simulink model "OPENXWD"  (R2022b)
settings: Solver=ode45  StartTime=0.0  StopTime=inf  RelTol=1e-3  EnableMultiTasking=on
PreLoadFcn:
  | run('Parameters\FSE_Parameters.m')
model workspace (MAT data in the model file):
  socvcb : containers.Map (value not decoded)
undefined symbols (not defined in the file): i_Diff
libraries: CarMaker4SL x21, simulink x16, eeGeneralControl x6
(part 5 of 8)

== system OPENXWD/CarMaker/IPG Vehicle/PowerTrain/Electric Powertrain/E-Gas // E-Motor/Subsystem1/VDC/Vehicle Dynamics Control Modes/VDC Complete/Optimization SKF & CKF ==
  RPM_INV1 : Inport
  RPM_INV2 : Inport  Port=2
  Steer_An : Inport  Port=3
  SKF_Initial : Inport  Port=4
  CKF_Initial : Inport  Port=5
  Cte_SKF : Inport  Port=6
  Cte_CKF : Inport  Port=7
  CKF_prev : DataStoreRead  DataStoreName=B  IndexOptions=Index vector (dialog)  Indices=1  OutputSizes=1
  Constant : Constant  Value=0
  Data Store Memory : DataStoreMemory  ReadBeforeWriteMsg=warning  WriteAfterWriteMsg=warning  WriteAfterReadMsg=warning  ShowAdditionalParam=off
  Data Store Memory1 : DataStoreMemory  DataStoreName=B  ReadBeforeWriteMsg=warning  WriteAfterWriteMsg=warning  WriteAfterReadMsg=warning  ShowAdditionalParam=off
  Data Store Write : DataStoreWrite  IndexOptions=Index vector (dialog)  Indices=1  OutputSizes=1
  Data Store Write1 : DataStoreWrite  DataStoreName=B  IndexOptions=Index vector (dialog)  Indices=1  OutputSizes=1
  Derivative : Derivative
  Display : Display
  Display1 : Display
  Display2 : Display
  MATLAB Function : MATLAB Function  TreatAsAtomicUnit=on
  Mux : Mux  Inputs=3
  "SKF_prev " : DataStoreRead  IndexOptions=Index vector (dialog)  Indices=1  OutputSizes=1
  Saturation : Saturate  UpperLimit=6000  LowerLimit=0
  Scope : Scope
  "Subsystem " : Subsystem
  Switch : Switch  Threshold=900  SaturateOnIntegerOverflow=off  InputSameDT=off
  SKF_act : Outport  VectorParamsAs1DForOutWhenUnconnected=off
  CKF_act : Outport  Port=2  VectorParamsAs1DForOutWhenUnconnected=off
  wires:
  SKF_Initial/1 -> "Subsystem "/3(SKF_Initial)
  CKF_prev/1 -> "Subsystem "/6("CKF_prev ")
  "Subsystem "/1("SKF_act ") -> SKF_act/1, Display1/1, Data Store Write/1  "SKF"
  Derivative/1 -> Switch/1, Switch/2, Saturation/1, Display/1, "Subsystem "/2(Derivative)  "alpha"
  "SKF_prev "/1 -> "Subsystem "/4(SKF_prev)
  "Subsystem "/2(CKF_act) -> CKF_act/1, Display2/1, Data Store Write1/1  "CKF"
  Cte_CKF/1 -> "Subsystem "/8(Cte_CKF)
  Steer_An/1 -> "Subsystem "/1(Steer_An)
  CKF_Initial/1 -> "Subsystem "/5("CKF_Initial ")
  Cte_SKF/1 -> "Subsystem "/7(Cte_SKF)
  MATLAB Function/1(RPM) -> Derivative/1  "w (rad/s)"
  Mux/1 -> Scope/1
  Saturation/1 -> Mux/2
  Switch/1 -> Mux/3
  Constant/1 -> Switch/3
  RPM_INV1/1 -> Mux/1, MATLAB Function/1(RPM_INV1)
  RPM_INV2/1 -> MATLAB Function/2(RPM_INV2)

== system OPENXWD/CarMaker/IPG Vehicle/PowerTrain/Electric Powertrain/E-Gas // E-Motor/Subsystem1/VDC/Vehicle Dynamics Control Modes/VDC Complete/Sensor_DATA ==
  note: [deg]
  note: [N]
  note: [N]
  note: [N]
  note: [N]
  note: [0-1]
  note: [0-1]
  note: [0 or 1]
  note: [rad/s]
  note: [rad/s]
  note: [rad/s]
  note: [m/s2]
  note: [m/s]
  Steer_Ang : Inport
  Ellipse_acc : Inport  Port=2
  Gyro_Ellipse : Inport  Port=3
  FR_Susp : Inport  Port=4
  FL_Susp : Inport  Port=5
  RR_Susp : Inport  Port=6
  RL_Susp : Inport  Port=7
  Gas Pedal : Inport  Port=8
  Brake Pedal : Inport  Port=9
  Regenerative Enable : Inport  Port=10
  V_eRR : Inport  Port=11
  "V_eRL " : Inport  Port=12
  Ellipse_vel : Inport  Port=13
  Steer_ang : Outport  VectorParamsAs1DForOutWhenUnconnected=off
  Ellipse_Acc : Outport  Port=2  VectorParamsAs1DForOutWhenUnconnected=off
  GyroEllipse : Outport  Port=3  VectorParamsAs1DForOutWhenUnconnected=off
  FR_susp : Outport  Port=4  VectorParamsAs1DForOutWhenUnconnected=off
  FL_susp : Outport  Port=5  VectorParamsAs1DForOutWhenUnconnected=off
  RR_susp : Outport  Port=6  VectorParamsAs1DForOutWhenUnconnected=off
  RL_susp : Outport  Port=7  VectorParamsAs1DForOutWhenUnconnected=off
  Gas_Pedal : Outport  Port=8  VectorParamsAs1DForOutWhenUnconnected=off
  Brake_Pedal : Outport  Port=9  VectorParamsAs1DForOutWhenUnconnected=off
  Reg_Enable : Outport  Port=10  VectorParamsAs1DForOutWhenUnconnected=off
  "V_eRR " : Outport  Port=11  VectorParamsAs1DForOutWhenUnconnected=off
  V_eRL : Outport  Port=12  VectorParamsAs1DForOutWhenUnconnected=off
  Ellipse_Vel : Outport  Port=13
  wires:
  RL_Susp/1 -> RL_susp/1
  RR_Susp/1 -> RR_susp/1
  FL_Susp/1 -> FL_susp/1
  FR_Susp/1 -> FR_susp/1
  Steer_Ang/1 -> Steer_ang/1
  Gas Pedal/1 -> Gas_Pedal/1
  Brake Pedal/1 -> Brake_Pedal/1
  Regenerative Enable/1 -> Reg_Enable/1
  "V_eRL "/1 -> V_eRL/1
  V_eRR/1 -> "V_eRR "/1
  Gyro_Ellipse/1 -> GyroEllipse/1
  Ellipse_acc/1 -> Ellipse_Acc/1
  Ellipse_vel/1 -> Ellipse_Vel/1

== system OPENXWD/CarMaker/IPG Vehicle/PowerTrain/Electric Powertrain/E-Gas // E-Motor/Subsystem1/VDC/Vehicle Dynamics Control Modes/VDC Complete/Wheel_to_motor ==
  "Fx_FR " : Inport
  "Fx_FL " : Inport  Port=2
  "Fx_RR " : Inport  Port=3
  "Fx_RL " : Inport  Port=4
  Re : Inport  Port=5
  RT : Inport  Port=6
  Add : Sum  Inputs=+-
  Constant : Constant  Value=0
  Constant1 : Constant  Value=0
  Fx_to_engineTqRL : Subsystem
  Fx_to_engineTqRR : Subsystem
  MATLAB Function1 : MATLAB Function  TreatAsAtomicUnit=on
  MATLAB Function2 : MATLAB Function  TreatAsAtomicUnit=on
  Tq_diff : Outport
  Tq_FR : Outport  Port=2  VectorParamsAs1DForOutWhenUnconnected=off
  Tq_FL : Outport  Port=3  VectorParamsAs1DForOutWhenUnconnected=off
  Tq_RR : Outport  Port=4  VectorParamsAs1DForOutWhenUnconnected=off
  Tq_RL : Outport  Port=5  VectorParamsAs1DForOutWhenUnconnected=off
  wires:
  Fx_to_engineTqRR/1(Tq) -> Add/1, Tq_RR/1
  Fx_to_engineTqRL/1(Tq) -> Tq_RL/1, Add/2
  "Fx_FR "/1 -> Tq_FR/1
  "Fx_FL "/1 -> Tq_FL/1
  Re/1 -> Fx_to_engineTqRR/2(Re), Fx_to_engineTqRL/2(Re)
  RT/1 -> Fx_to_engineTqRR/3(RT), Fx_to_engineTqRL/3(RT)
  "Fx_RL "/1 -> MATLAB Function2/2(v)
  "Fx_RR "/1 -> MATLAB Function1/2(v)
  MATLAB Function2/1(value) -> Fx_to_engineTqRL/1(Fx)
  MATLAB Function1/1(value) -> Fx_to_engineTqRR/1(Fx)
  Constant1/1 -> MATLAB Function1/1(cte)
  Constant/1 -> MATLAB Function2/1(cte)
  Add/1 -> Tq_diff/1

== system OPENXWD/CarMaker/IPG Vehicle/PowerTrain/Electric Powertrain/E-Gas // E-Motor/Subsystem1/VDC/Vehicle Dynamics Control Modes/VDC without Longitudinal/Constraints ==
  Tq_FRin : Inport
  Tq_FLin : Inport  Port=2
  Tq_RR_wc : Inport  Port=3
  "Tq_RL_wc " : Inport  Port=4
  "Trans_max_static " : Inport  Port=5
  Trans_max_dynamic : Inport  Port=6
  V_eRR : Inport  Port=7
  V_eRL : Inport  Port=8
  Tq_max : Inport  Port=9
  MaxRegTorque : Inport  Port=10
  Bp : Inport  Port=11
  Reg_enable : Inport  Port=12
  RT : Inport  Port=13
  Acelerating and braking without Regenerative : Subsystem  TreatAsAtomicUnit=on
  Braking with Regenerative : Subsystem  TreatAsAtomicUnit=on
  Constant : Constant  Value=0
  Constant1 : Constant  Value=0
  If : If  NumInputs=2  IfExpression=u2 == 1 & u1 > 0
  Merge1 : Merge
  Merge2 : Merge
  Tq_FRout : Outport  VectorParamsAs1DForOutWhenUnconnected=off
  "Tq_FLout " : Outport  Port=2  VectorParamsAs1DForOutWhenUnconnected=off
  Tq_RRout : Outport  Port=3  VectorParamsAs1DForOutWhenUnconnected=off
  Tq_RLout : Outport  Port=4  VectorParamsAs1DForOutWhenUnconnected=off
  wires:
  Constant1/1 -> "Tq_FLout "/1
  Constant/1 -> Tq_FRout/1
  Tq_RR_wc/1 -> Acelerating and braking without Regenerative/9(Tq_RR), Braking with Regenerative/2(Tq_RR_wc)
  "Tq_RL_wc "/1 -> Braking with Regenerative/3(Tq_RL_wc), Acelerating and braking without Regenerative/10(Tq_RL)
  Tq_max/1 -> Acelerating and braking without Regenerative/2(Tq_max)
  V_eRL/1 -> Acelerating and braking without Regenerative/4(V_eRL)
  Trans_max_dynamic/1 -> Acelerating and braking without Regenerative/5(Trans_dynamic_max_motor_Tq)
  "Trans_max_static "/1 -> Acelerating and braking without Regenerative/6(Trans_static_max_motor_Tq)
  Merge2/1 -> Tq_RLout/1
  Merge1/1 -> Tq_RRout/1
  Bp/1 -> If/1
  Reg_enable/1 -> If/2
  V_eRR/1 -> Acelerating and braking without Regenerative/3(V_eRR)
  If/1 -> Braking with Regenerative/Action
  If/2 -> Acelerating and braking without Regenerative/Action
  MaxRegTorque/1 -> Braking with Regenerative/1(MaxRegTorque)
  Tq_FRin/1 -> Acelerating and braking without Regenerative/7(Tq_FR)
  Tq_FLin/1 -> Acelerating and braking without Regenerative/8(Tq_FL)
  Acelerating and braking without Regenerative/2(TQ_RL) -> Merge2/1
  Acelerating and braking without Regenerative/1(TQ_RR) -> Merge1/1
  Braking with Regenerative/1(TQ_RR) -> Merge1/2
  Braking with Regenerative/2(TQ_RL) -> Merge2/2
  RT/1 -> Acelerating and braking without Regenerative/1(Transmission Ratio)

== system OPENXWD/CarMaker/IPG Vehicle/PowerTrain/Electric Powertrain/E-Gas // E-Motor/Subsystem1/VDC/Vehicle Dynamics Control Modes/VDC without Longitudinal/Driver // CarBehaviours ==
  Tq_FRin : Inport
  Tq_FLin : Inport  Port=2
  Tq_RRin : Inport  Port=3
  "Tq_RLin " : Inport  Port=4
  Bp : Inport  Port=5
  Ap : Inport  Port=6
  Reg_enable : Inport  Port=7
  Ap_Sat_up : Inport  Port=8
  Ap_Sat_down : Inport  Port=9
  Accelerating : Subsystem  TreatAsAtomicUnit=on
  Braking Conditions : If  NumInputs=4  IfExpression=u1>0.2 & u2<=u4 & u3==1  ElseIfExpressions=u1>0.2 & u2<=u4 & u3==0, u1==0 & u2==0
  Constant : Constant  Value=0
  Constant1 : Constant  Value=0
  Inertia Braking : Subsystem  TreatAsAtomicUnit=on
  Mech_Braking : Subsystem  TreatAsAtomicUnit=on
  Merge : Merge  Inputs=4
  Merge1 : Merge  Inputs=4
  Regenerative+Mech Braking : Subsystem  TreatAsAtomicUnit=on
  Terminator : Terminator
  Terminator1 : Terminator
  Tq_FRout : Outport  VectorParamsAs1DForOutWhenUnconnected=off
  "Tq_FLout " : Outport  Port=2  VectorParamsAs1DForOutWhenUnconnected=off
  Tq_RRout : Outport  Port=3  VectorParamsAs1DForOutWhenUnconnected=off
  Tq_RLout : Outport  Port=4  VectorParamsAs1DForOutWhenUnconnected=off
  out_Throttle : Outport  Port=5  VectorParamsAs1DForOutWhenUnconnected=off
  wires:
  Constant1/1 -> "Tq_FLout "/1
  Constant/1 -> Tq_FRout/1
  Tq_FLin/1 -> Terminator1/1
  Tq_FRin/1 -> Terminator/1
  Merge/1 -> Tq_RRout/1
  Merge1/1 -> Tq_RLout/1
  Bp/1 -> Regenerative+Mech Braking/1(Bp), Braking Conditions/1
  Ap/1 -> Accelerating/1(Ap), Braking Conditions/2
  Regenerative+Mech Braking/1("Tq_RR ") -> Merge/1
  Mech_Braking/1("Tq_RR ") -> Merge/2
  Inertia Braking/1("Tq_RR ") -> Merge/3
  Accelerating/1("Tq_RR ") -> Merge/4
  Regenerative+Mech Braking/2(Tq_RL) -> Merge1/1
  Mech_Braking/2(Tq_RL) -> Merge1/2
  Inertia Braking/2(Tq_RL) -> Merge1/3
  Accelerating/2(Tq_RL) -> Merge1/4
  Braking Conditions/1 -> Regenerative+Mech Braking/Action
  Braking Conditions/2 -> Mech_Braking/Action
  Braking Conditions/3 -> Inertia Braking/Action
  Braking Conditions/4 -> Accelerating/Action
  Tq_RRin/1 -> Regenerative+Mech Braking/2(Tq_max_RR), Accelerating/4(Tq_RR)
  "Tq_RLin "/1 -> Regenerative+Mech Braking/3(Tq_max_RL), Accelerating/5("Tq_RL ")
  Ap_Sat_up/1 -> Accelerating/2("Ap_Sat_up ")
  Ap_Sat_down/1 -> Accelerating/3(Ap_Sat_down), Braking Conditions/4
  Reg_enable/1 -> Braking Conditions/3
  Accelerating/3(Out_Throttle) -> out_Throttle/1

== system OPENXWD/CarMaker/IPG Vehicle/PowerTrain/Electric Powertrain/E-Gas // E-Motor/Subsystem1/VDC/Vehicle Dynamics Control Modes/VDC without Longitudinal/Force to Tq ==
  "Fx_FR " : Inport
  "Fx_FL " : Inport  Port=2
  "Fx_RR " : Inport  Port=3
  "Fx_RL " : Inport  Port=4
  Re : Inport  Port=5
  Constant : Constant  Value=0
  Constant1 : Constant  Value=0
  Fx_to_wheelTqRL : Subsystem
  Fx_to_wheelTqRR : Subsystem
  MATLAB Function1 : MATLAB Function  TreatAsAtomicUnit=on
  MATLAB Function2 : MATLAB Function  TreatAsAtomicUnit=on
  Tq_FR : Outport  VectorParamsAs1DForOutWhenUnconnected=off
  Tq_FL : Outport  Port=2  VectorParamsAs1DForOutWhenUnconnected=off
  Tq_RR : Outport  Port=3  VectorParamsAs1DForOutWhenUnconnected=off
  Tq_RL : Outport  Port=4  VectorParamsAs1DForOutWhenUnconnected=off
  wires:
  Fx_to_wheelTqRR/1(Tq) -> Tq_RR/1
  Fx_to_wheelTqRL/1(Tq) -> Tq_RL/1
  "Fx_FR "/1 -> Tq_FR/1
  "Fx_FL "/1 -> Tq_FL/1
  Re/1 -> Fx_to_wheelTqRR/2(Re), Fx_to_wheelTqRL/2(Re)
  "Fx_RR "/1 -> MATLAB Function2/2(v)
  "Fx_RL "/1 -> MATLAB Function1/2(v)
  MATLAB Function2/1(value) -> Fx_to_wheelTqRR/1(Fx)
  Constant/1 -> MATLAB Function2/1(cte)
  Constant1/1 -> MATLAB Function1/1(cte)
  MATLAB Function1/1(value) -> Fx_to_wheelTqRL/1(Fx)

== system OPENXWD/CarMaker/IPG Vehicle/PowerTrain/Electric Powertrain/E-Gas // E-Motor/Subsystem1/VDC/Vehicle Dynamics Control Modes/VDC without Longitudinal/In_Numbers ==
  C-Kamm_Factor : Inport
  Max Regen Torque [Nm] : Inport  Port=2
  Steering Saturation (per site) [deg] : Inport  Port=3
  Ap_Sat_Down [-] : Inport  Port=4
  Ap_Sat_Up [-] : Inport  Port=5
  3% difference : Gain  Gain=0.97
  Diameter to Radius : Gain  Gain=1/2
  Effective Rolling Diameter[inch] : Constant  Value=18
  Engine+Inverter Performance [-] : Constant  Value=0.8
  Maximum Torque per motor [Nm] : Constant  Value=120
  Maximum Transmission Torque Dynamic [Nm] : Constant  Value=140
  Maximum Transmission Torque Static [Nm] : Constant  Value=130
  Product : Product
  Transmision Ratio[-] : Constant  Value=4
  inch to m : Gain  Gain=0.0254
  Steer_Sat [deg] : Outport  VectorParamsAs1DForOutWhenUnconnected=off
  Tq_Max_Wheel [Nm] : Outport  Port=2  VectorParamsAs1DForOutWhenUnconnected=off
  Cornering Kamm_Factor [0-2] : Outport  Port=3  VectorParamsAs1DForOutWhenUnconnected=off
  Transmision_Ratio[-] : Outport  Port=4  VectorParamsAs1DForOutWhenUnconnected=off
  Effective Rolling Radius[m] : Outport  Port=5  VectorParamsAs1DForOutWhenUnconnected=off
  Ap_Sat_down[-] : Outport  Port=6  VectorParamsAs1DForOutWhenUnconnected=off
  Ap_Sat_up[-] : Outport  Port=7  VectorParamsAs1DForOutWhenUnconnected=off
  Engine+Inverter Performance[-] : Outport  Port=8  VectorParamsAs1DForOutWhenUnconnected=off
  Trans_max _static[Nm] : Outport  Port=9  VectorParamsAs1DForOutWhenUnconnected=off
  Trans_max_dynamic [Nm] : Outport  Port=10  VectorParamsAs1DForOutWhenUnconnected=off
  MaxRegTorque [Nm] : Outport  Port=11  VectorParamsAs1DForOutWhenUnconnected=off
  wires:
  Transmision Ratio[-]/1 -> Product/2, Transmision_Ratio[-]/1
  Effective Rolling Diameter[inch]/1 -> Diameter to Radius/1
  Maximum Transmission Torque Static [Nm]/1 -> Trans_max _static[Nm]/1
  Maximum Transmission Torque Dynamic [Nm]/1 -> Trans_max_dynamic [Nm]/1
  inch to m/1 -> 3% difference/1
  3% difference/1 -> Effective Rolling Radius[m]/1
  Engine+Inverter Performance [-]/1 -> Engine+Inverter Performance[-]/1
  Max Regen Torque [Nm]/1 -> MaxRegTorque [Nm]/1
  C-Kamm_Factor/1 -> Cornering Kamm_Factor [0-2]/1
  Steering Saturation (per site) [deg]/1 -> Steer_Sat [deg]/1
  Ap_Sat_Up [-]/1 -> Ap_Sat_up[-]/1
  Ap_Sat_Down [-]/1 -> Ap_Sat_down[-]/1
  Diameter to Radius/1 -> inch to m/1
  Product/1 -> Tq_Max_Wheel [Nm]/1
  Maximum Torque per motor [Nm]/1 -> Product/1

== system OPENXWD/CarMaker/IPG Vehicle/PowerTrain/Electric Powertrain/E-Gas // E-Motor/Subsystem1/VDC/Vehicle Dynamics Control Modes/VDC without Longitudinal/Kamm Circle Lateral ==
  "N_FR " : Inport
  N_FL : Inport  Port=2
  N_RR : Inport  Port=3
  N_RL : Inport  Port=4
  Fy : Inport  Port=5
  CK_Factor : Inport  Port=6
  Constant : Constant  Value=-1
  Constant1 : Constant  Value=-1
  Kamm_Circle LatD : MATLAB Function  TreatAsAtomicUnit=on
  MATLAB Function1 : MATLAB Function  TreatAsAtomicUnit=on
  MATLAB Function2 : MATLAB Function  TreatAsAtomicUnit=on
  Product : Product
  Product1 : Product
  Fx_FR : Outport  VectorParamsAs1DForOutWhenUnconnected=off
  Fx_FL : Outport  Port=2  VectorParamsAs1DForOutWhenUnconnected=off
  "Fx_RR " : Outport  Port=3  VectorParamsAs1DForOutWhenUnconnected=off
  "Fx_RL " : Outport  Port=4  VectorParamsAs1DForOutWhenUnconnected=off
  wires:
  N_FL/1 -> Fx_FL/1
  "N_FR "/1 -> Fx_FR/1
  N_RL/1 -> Kamm_Circle LatD/2(Fz_L)
  Fy/1 -> Kamm_Circle LatD/3(Fy)
  N_RR/1 -> Kamm_Circle LatD/1(Fz_R)
  Kamm_Circle LatD/1(Fx_R) -> Product/1
  Kamm_Circle LatD/2(Fx_L) -> Product1/1
  CK_Factor/1 -> Product/2, Product1/2
  Product1/1 -> MATLAB Function1/2(v)
  Product/1 -> MATLAB Function2/2(v)
  Constant1/1 -> MATLAB Function2/1(cte)
  Constant/1 -> MATLAB Function1/1(cte)
  MATLAB Function2/1(value) -> "Fx_RR "/1
  MATLAB Function1/1(value) -> "Fx_RL "/1

== system OPENXWD/CarMaker/IPG Vehicle/PowerTrain/Electric Powertrain/E-Gas // E-Motor/Subsystem1/VDC/Vehicle Dynamics Control Modes/VDC without Longitudinal/Lateral Dynamics ==
  FR_susp : Inport
  FL_susp : Inport  Port=2
  RR_susp : Inport  Port=3
  RL_susp : Inport  Port=4
  Gas_pedal : Inport  Port=5
  Brake_pedal : Inport  Port=6
  Ellipse_acc : Inport  Port=7
  Constant : Constant  Value=0
  Constant1 : Constant  Value=0
  Constant2 : Constant  Value=0
  Demux : Demux  Outputs=3
  Fy per wheel : Gain  Gain=1/2
  Gravity : Gain  Gain=1/9.81
  Gravity1 : Gain  Gain=1/9.81
  Product : Product
  Sum : Sum  Inputs=++++
  Sum1 : Sum
  Terminator{3..6} (4 alike) : Terminator
  N_FR : Outport  VectorParamsAs1DForOutWhenUnconnected=off
  "N_FL " : Outport  Port=2  VectorParamsAs1DForOutWhenUnconnected=off
  "N_RR " : Outport  Port=3  VectorParamsAs1DForOutWhenUnconnected=off
  N_RL : Outport  Port=4  VectorParamsAs1DForOutWhenUnconnected=off
  Fy_R : Outport  Port=5  VectorParamsAs1DForOutWhenUnconnected=off
  Mass [kg] (0,inf) : Outport  Port=6  VectorParamsAs1DForOutWhenUnconnected=off
  Handling [-] (-inf,inf) : Outport  Port=7  VectorParamsAs1DForOutWhenUnconnected=off
  wires:
  Constant2/1 -> "N_FL "/1
  Constant1/1 -> N_FR/1
  Gas_pedal/1 -> Terminator4/1
  Brake_pedal/1 -> Terminator5/1
  Demux/2 -> Product/1
  Demux/1 -> Terminator6/1
  Demux/3 -> Terminator3/1
  Product/1 -> Fy per wheel/1  "Fy per axe"
  Fy per wheel/1 -> Fy_R/1
  Gravity1/1 -> Product/2
  Sum/1 -> Gravity/1
  Sum1/1 -> Gravity1/1
  Gravity/1 -> Mass [kg] (0,inf)/1  "Mass [kg]"
  RL_susp/1 -> N_RL/1, Sum1/2, Sum/4
  RR_susp/1 -> Sum1/1, "N_RR "/1, Sum/3
  FL_susp/1 -> Sum/2
  FR_susp/1 -> Sum/1
  Ellipse_acc/1 -> [ellipse_acc]
  Constant/1 -> Handling [-] (-inf,inf)/1
  [ellipse_acc] -> Demux/1

== system OPENXWD/CarMaker/IPG Vehicle/PowerTrain/Electric Powertrain/E-Gas // E-Motor/Subsystem1/VDC/Vehicle Dynamics Control Modes/VDC without Longitudinal/Optimization SKF & CKF ==
  RPM_INV1 : Inport
  RPM_INV2 : Inport  Port=2
  CKF_Initial : Inport  Port=3
  Cte_CKF : Inport  Port=4
  CKF_prev : DataStoreRead  DataStoreName=B  IndexOptions=Index vector (dialog)  Indices=1  OutputSizes=1
  Data Store Memory1 : DataStoreMemory  DataStoreName=B  ReadBeforeWriteMsg=warning  WriteAfterWriteMsg=warning  WriteAfterReadMsg=warning  ShowAdditionalParam=off
  Data Store Write1 : DataStoreWrite  DataStoreName=B  IndexOptions=Index vector (dialog)  Indices=1  OutputSizes=1
  Derivative : Derivative
  MATLAB Function : MATLAB Function  TreatAsAtomicUnit=on
  "Subsystem " : Subsystem
  CKF_act : Outport  VectorParamsAs1DForOutWhenUnconnected=off
  wires:
  CKF_prev/1 -> "Subsystem "/3("CKF_prev ")
  Derivative/1 -> "Subsystem "/1(Derivative)  "alpha"
  MATLAB Function/1(RPM) -> Derivative/1  "w (rad/s)"
  "Subsystem "/1(CKF_act) -> Data Store Write1/1, CKF_act/1  "CKF"
  Cte_CKF/1 -> "Subsystem "/4(Cte_CKF)
  CKF_Initial/1 -> "Subsystem "/2("CKF_Initial ")
  RPM_INV1/1 -> MATLAB Function/1(RPM_INV1)
  RPM_INV2/1 -> MATLAB Function/2(RPM_INV2)

== system OPENXWD/CarMaker/IPG Vehicle/PowerTrain/Electric Powertrain/E-Gas // E-Motor/Subsystem1/VDC/Vehicle Dynamics Control Modes/VDC without Longitudinal/Sensor_DATA ==
  note: [deg]
  note: [N]
  note: [N]
  note: [N]
  note: [N]
  note: [0-1]
  note: [0-1]
  note: [0 or 1]
  note: [rad/s]
  note: [rad/s]
  note: [m/s2]
  Steer_Ang : Inport
  FR_Susp : Inport  Port=2
  FL_Susp : Inport  Port=3
  RR_Susp : Inport  Port=4
  RL_Susp : Inport  Port=5
  Gas Pedal : Inport  Port=6
  Brake Pedal : Inport  Port=7
  Regenerative Enable : Inport  Port=8
  V_eRR : Inport  Port=9
  "V_eRL " : Inport  Port=10
  Ellipse_acc_ax_ay_az : Inport  Port=11
  Steer_ang : Outport  VectorParamsAs1DForOutWhenUnconnected=off
  FR_susp : Outport  Port=2  VectorParamsAs1DForOutWhenUnconnected=off
  FL_susp : Outport  Port=3  VectorParamsAs1DForOutWhenUnconnected=off
  RR_susp : Outport  Port=4  VectorParamsAs1DForOutWhenUnconnected=off
  RL_susp : Outport  Port=5  VectorParamsAs1DForOutWhenUnconnected=off
  Gas_Pedal : Outport  Port=6  VectorParamsAs1DForOutWhenUnconnected=off
  Brake_Pedal : Outport  Port=7  VectorParamsAs1DForOutWhenUnconnected=off
  Reg_Enable : Outport  Port=8  VectorParamsAs1DForOutWhenUnconnected=off
  "V_eRR " : Outport  Port=9  VectorParamsAs1DForOutWhenUnconnected=off
  V_eRL : Outport  Port=10  VectorParamsAs1DForOutWhenUnconnected=off
  Ellipse_acc : Outport  Port=11  VectorParamsAs1DForOutWhenUnconnected=off
  wires:
  RL_Susp/1 -> RL_susp/1
  RR_Susp/1 -> RR_susp/1
  FL_Susp/1 -> FL_susp/1
  FR_Susp/1 -> FR_susp/1
  Steer_Ang/1 -> Steer_ang/1
  Gas Pedal/1 -> Gas_Pedal/1
  Brake Pedal/1 -> Brake_Pedal/1
  Regenerative Enable/1 -> Reg_Enable/1
  "V_eRL "/1 -> V_eRL/1
  V_eRR/1 -> "V_eRR "/1
  Ellipse_acc_ax_ay_az/1 -> Ellipse_acc/1

== system OPENXWD/CarMaker/IPG Vehicle/PowerTrain/Electric Powertrain/E-Gas // E-Motor/Subsystem1/VDC/Vehicle Dynamics Control Modes/Steering TV with TC/Accelerating, Braking or Regen Braking/Accelerating ==
  Throttle : Inport
  Tq_RR : Inport  Port=2
  "Tq_RL " : Inport  Port=3
  Action Port : ActionPort  ActionPortLabel=else
  Product : Product
  Product1 : Product
  "Tq_RR " : Outport  VectorParamsAs1DForOutWhenUnconnected=off
  Tq_RL : Outport  Port=2  VectorParamsAs1DForOutWhenUnconnected=off
  wires:
  Product1/1 -> "Tq_RR "/1
  Product/1 -> Tq_RL/1
  Throttle/1 -> Product/1, Product1/1
  Tq_RR/1 -> Product1/2
  "Tq_RL "/1 -> Product/2

== system OPENXWD/CarMaker/IPG Vehicle/PowerTrain/Electric Powertrain/E-Gas // E-Motor/Subsystem1/VDC/Vehicle Dynamics Control Modes/Steering TV with TC/Accelerating, Braking or Regen Braking/Inertia Braking ==
  Action Port : ActionPort  ActionPortLabel=elseif( u1<=0.2 & u2<=0)
  Constant : Constant  Value=0
  Constant1 : Constant  Value=0
  "Tq_RR " : Outport  VectorParamsAs1DForOutWhenUnconnected=off
  Tq_RL : Outport  Port=2  VectorParamsAs1DForOutWhenUnconnected=off
  wires:
  Constant1/1 -> Tq_RL/1
  Constant/1 -> "Tq_RR "/1

== system OPENXWD/CarMaker/IPG Vehicle/PowerTrain/Electric Powertrain/E-Gas // E-Motor/Subsystem1/VDC/Vehicle Dynamics Control Modes/Steering TV with TC/Accelerating, Braking or Regen Braking/Mech_Braking ==
  Action Port : ActionPort  ActionPortLabel=elseif(u1>0.2 & u2<=0 & u3==0)
  Constant : Constant  Value=0
  Constant1 : Constant  Value=0
  "Tq_RR " : Outport  VectorParamsAs1DForOutWhenUnconnected=off
  Tq_RL : Outport  Port=2  VectorParamsAs1DForOutWhenUnconnected=off
  wires:
  Constant1/1 -> Tq_RL/1
  Constant/1 -> "Tq_RR "/1

== system OPENXWD/CarMaker/IPG Vehicle/PowerTrain/Electric Powertrain/E-Gas // E-Motor/Subsystem1/VDC/Vehicle Dynamics Control Modes/Steering TV with TC/Accelerating, Braking or Regen Braking/Regenerative+Mech Braking ==
  Max_Regen_Tq : Inport
  Bp : Inport  Port=2
  RegTq_RR : Inport  Port=3
  RegTq_RL : Inport  Port=4
  Action Port : ActionPort  ActionPortLabel=if(u1>0.2 & u2<=0 & u3==1)
  Gain : Gain  Gain=-1
  Gain1 : Gain  Gain=-1
  MATLAB Function : MATLAB Function  TreatAsAtomicUnit=on
  MATLAB Function1 : MATLAB Function  TreatAsAtomicUnit=on
  "Tq_RR " : Outport  VectorParamsAs1DForOutWhenUnconnected=off
  Tq_RL : Outport  Port=2  VectorParamsAs1DForOutWhenUnconnected=off
  wires:
  MATLAB Function1/1(RegTq_RR) -> Gain/1
  Gain/1 -> "Tq_RR "/1
  Gain1/1 -> Tq_RL/1
  MATLAB Function1/2(RegTq_RL) -> Gain1/1
  MATLAB Function/2(Tq_regen_RL) -> MATLAB Function1/3(Tq_RL)
  MATLAB Function/1(Tq_regen_RR) -> MATLAB Function1/2(Tq_RR)
  Bp/1 -> MATLAB Function/1(Bp)
  RegTq_RR/1 -> MATLAB Function/2(Tq_max_RR)
  RegTq_RL/1 -> MATLAB Function/3(Tq_max_RL)
  Max_Regen_Tq/1 -> MATLAB Function1/1(MaxRegenTq)

== system OPENXWD/CarMaker/IPG Vehicle/PowerTrain/Electric Powertrain/E-Gas // E-Motor/Subsystem1/VDC/Vehicle Dynamics Control Modes/Steering TV with TC/Optimization SKF & CKF/Subsystem  ==
  Steer_An : Inport
  Derivative : Inport  Port=2
  SKF_Initial : Inport  Port=3
  SKF_prev : Inport  Port=4
  "CKF_Initial " : Inport  Port=5
  "CKF_prev " : Inport  Port=6
  Cte_SKF : Inport  Port=7
  Cte_CKF : Inport  Port=8
  CKF : Subsystem
  MATLAB Function1 : MATLAB Function  TreatAsAtomicUnit=on
  SKF : Subsystem
  SKF or CKF : If  IfExpression=-10 < u1 & u1 < 10
  Steering Wheel Maximum Angle : Constant  Value=100
  "SKF_act " : Outport  VectorParamsAs1DForOutWhenUnconnected=off
  CKF_act : Outport  Port=2  VectorParamsAs1DForOutWhenUnconnected=off
  wires:
  MATLAB Function1/1(value) -> SKF or CKF/1
  Steering Wheel Maximum Angle/1 -> MATLAB Function1/1(cte)
  Steer_An/1 -> MATLAB Function1/2(v)
  SKF/1(SKF_act) -> "SKF_act "/1
  CKF/1("CKF_act ") -> CKF_act/1
  SKF or CKF/1 -> SKF/Action
  SKF or CKF/2 -> CKF/Action
  "CKF_prev "/1 -> CKF/3("CKF_prev ")
  Derivative/1 -> CKF/1(Derivative), SKF/1(Derivative)
  SKF_Initial/1 -> SKF/2("SKF_Initial ")
  SKF_prev/1 -> SKF/3(SKF_prev)
  "CKF_Initial "/1 -> CKF/2(CKF_Initial)
  Cte_SKF/1 -> SKF/4(Cte_SKF)
  Cte_CKF/1 -> CKF/4(Cte_CKF)

== system OPENXWD/CarMaker/IPG Vehicle/PowerTrain/Electric Powertrain/E-Gas // E-Motor/Subsystem1/VDC/Vehicle Dynamics Control Modes/VDC Complete/Constraints and motor to wheel Tq/Acelerating and braking without Regenerative ==
  note: Tq_lim y Flag_Power: antiguamente había aquí la limitación por temperatura y potencia
  Tq_max : Inport
  V_eRR : Inport  Port=2
  V_eRL : Inport  Port=3
  Trans_max_dynamic : Inport  Port=4
  Trans_max_static : Inport  Port=5
  Tq_FR : Inport  Port=6
  Tq_FL : Inport  Port=7
  Tq_RR : Inport  Port=8
  Tq_RL : Inport  Port=9
  Tq_diff : Inport  Port=10
  Tq_diff_max : Inport  Port=11
  Action Port : ActionPort  ActionPortLabel=else
  Constant : Constant  Value=0
  Gain : Gain  Gain=3.141592/30
  If Action 1 : Subsystem  TreatAsAtomicUnit=on
  If Action 2 : Subsystem  TreatAsAtomicUnit=on
  If1 : If  NumInputs=3  IfExpression=u1 > u3 & u2 > u3
  MATLAB Function : MATLAB Function  TreatAsAtomicUnit=on
  Merge2 : Merge
  Momentum Z scaled : Subsystem
  Terminator : Terminator
  Terminator1 : Terminator
  minimum value : MATLAB Function  TreatAsAtomicUnit=on
  minimum value1 : MATLAB Function  TreatAsAtomicUnit=on
  rpm : Constant  Value=200
  TQ_RR : Outport  VectorParamsAs1DForOutWhenUnconnected=off
  TQ_RL : Outport  Port=2  VectorParamsAs1DForOutWhenUnconnected=off
  Flag_Power : Outport  Port=3  VectorParamsAs1DForOutWhenUnconnected=off
  wires:
  If1/1 -> If Action 1/Action
  If Action 1/1(Trans_limit) -> Merge2/1
  Merge2/1 -> minimum value/1(a), minimum value1/1(a)
  Trans_max_dynamic/1 -> If Action 1/1(Trans_max_dynamic)
  If Action 2/1(Trans_limit) -> Merge2/2
  V_eRR/1 -> If1/1
  V_eRL/1 -> If1/2
  If1/2 -> If Action 2/Action
  Trans_max_static/1 -> If Action 2/1("Trans_max_static ")
  Tq_max/1 -> minimum value1/2(b), minimum value/2(b)
  rpm/1 -> Gain/1
  Gain/1 -> If1/3  "approx 20.95"
  Tq_FR/1 -> Terminator/1
  Tq_FL/1 -> Terminator1/1
  Tq_RR/1 -> [tq_RR_wc], minimum value/3(c)
  Tq_RL/1 -> [tq_RL_wc], minimum value1/3(c)
  [tq_RR_wc] -> Momentum Z scaled/3(Tq_RR_wc)
  [tq_RL_wc] -> Momentum Z scaled/4(Tq_RL_wc)
  Momentum Z scaled/1(TQ_RR) -> TQ_RR/1
  Momentum Z scaled/2(TQ_RL) -> TQ_RL/1
  Tq_diff/1 -> MATLAB Function/1(diff_wc)
  Tq_diff_max/1 -> MATLAB Function/2(diff_max)
  MATLAB Function/1(diff_lim) -> [Tq_diff_lim]
  [Tq_diff_lim] -> Momentum Z scaled/5(Tq_diff)
  minimum value/1(min) -> Momentum Z scaled/1(Tq_RR_Lim)
  minimum value1/1(min) -> Momentum Z scaled/2(Tq_RL_Lim)
  Constant/1 -> Flag_Power/1

== system OPENXWD/CarMaker/IPG Vehicle/PowerTrain/Electric Powertrain/E-Gas // E-Motor/Subsystem1/VDC/Vehicle Dynamics Control Modes/VDC Complete/Constraints and motor to wheel Tq/Braking with Regenerative ==
  MaxRegTorque : Inport
  Tq_RR_wc : Inport  Port=2
  Tq_RL_wc : Inport  Port=3
  Action Port : ActionPort  ActionPortLabel=if(u2 == 1 & u1 > 0)
  Gain : Gain  Gain=-1
  Gain1 : Gain  Gain=-1
  MATLAB Function : MATLAB Function  TreatAsAtomicUnit=on
  TQ_RR : Outport  VectorParamsAs1DForOutWhenUnconnected=off
  TQ_RL : Outport  Port=2  VectorParamsAs1DForOutWhenUnconnected=off
  wires:
  MaxRegTorque/1 -> MATLAB Function/1(MaxRegenTq)
  Gain1/1 -> TQ_RL/1
  Gain/1 -> TQ_RR/1
  MATLAB Function/1(RegTq_RR) -> Gain/1
  MATLAB Function/2(RegTq_RL) -> Gain1/1
  Tq_RL_wc/1 -> MATLAB Function/3(Tq_RL)
  Tq_RR_wc/1 -> MATLAB Function/2(Tq_RR)

== system OPENXWD/CarMaker/IPG Vehicle/PowerTrain/Electric Powertrain/E-Gas // E-Motor/Subsystem1/VDC/Vehicle Dynamics Control Modes/VDC Complete/Driver // CarBehaviours/Accelerating ==
  Throttle : Inport
  Tq_RR : Inport  Port=2
  "Tq_RL " : Inport  Port=3
  Action Port : ActionPort  ActionPortLabel=else
  Product : Product
  Product1 : Product
  "Tq_RR " : Outport  VectorParamsAs1DForOutWhenUnconnected=off
  Tq_RL : Outport  Port=2  VectorParamsAs1DForOutWhenUnconnected=off
  Out_Throttle : Outport  Port=3  VectorParamsAs1DForOutWhenUnconnected=off
  wires:
  Product1/1 -> "Tq_RR "/1
  Product/1 -> Tq_RL/1
  Throttle/1 -> Out_Throttle/1, Product/1, Product1/1
  Tq_RR/1 -> Product1/2
  "Tq_RL "/1 -> Product/2

== system OPENXWD/CarMaker/IPG Vehicle/PowerTrain/Electric Powertrain/E-Gas // E-Motor/Subsystem1/VDC/Vehicle Dynamics Control Modes/VDC Complete/Driver // CarBehaviours/Inertia Braking ==
  Action Port : ActionPort  ActionPortLabel=elseif( u1<0.1 & u2<0.1)
  Constant : Constant  Value=0
  Constant1 : Constant  Value=0
  "Tq_RR " : Outport  VectorParamsAs1DForOutWhenUnconnected=off
  Tq_RL : Outport  Port=2  VectorParamsAs1DForOutWhenUnconnected=off
  wires:
  Constant1/1 -> Tq_RL/1
  Constant/1 -> "Tq_RR "/1

== system OPENXWD/CarMaker/IPG Vehicle/PowerTrain/Electric Powertrain/E-Gas // E-Motor/Subsystem1/VDC/Vehicle Dynamics Control Modes/VDC Complete/Driver // CarBehaviours/Mech_Braking ==
  Action Port : ActionPort  ActionPortLabel=elseif(u1>0.2 & u2<0.1 & u3==0)
  Constant : Constant  Value=0
  Constant1 : Constant  Value=0
  "Tq_RR " : Outport  VectorParamsAs1DForOutWhenUnconnected=off
  Tq_RL : Outport  Port=2  VectorParamsAs1DForOutWhenUnconnected=off
  wires:
  Constant1/1 -> Tq_RL/1
  Constant/1 -> "Tq_RR "/1

== system OPENXWD/CarMaker/IPG Vehicle/PowerTrain/Electric Powertrain/E-Gas // E-Motor/Subsystem1/VDC/Vehicle Dynamics Control Modes/VDC Complete/Driver // CarBehaviours/Regenerative+Mech Braking ==
  Bp : Inport
  RegTq_RR : Inport  Port=2
  RegTq_RL : Inport  Port=3
  Action Port : ActionPort  ActionPortLabel=if(u1>0.2 & u2<0.1 & u3==1)
  MATLAB Function : MATLAB Function  TreatAsAtomicUnit=on
  "Tq_RR " : Outport  VectorParamsAs1DForOutWhenUnconnected=off
  Tq_RL : Outport  Port=2  VectorParamsAs1DForOutWhenUnconnected=off
  wires:
  RegTq_RR/1 -> MATLAB Function/2(Tq_max_RR)
  RegTq_RL/1 -> MATLAB Function/3(Tq_max_RL)
  MATLAB Function/1(Tq_regen_RR) -> "Tq_RR "/1
  Bp/1 -> MATLAB Function/1(Bp)
  MATLAB Function/2(Tq_regen_RL) -> Tq_RL/1

== system OPENXWD/CarMaker/IPG Vehicle/PowerTrain/Electric Powertrain/E-Gas // E-Motor/Subsystem1/VDC/Vehicle Dynamics Control Modes/VDC Complete/Lateral Dynamics/Kamm_Circle ==
  Fz_R : Inport
  Fz_L : Inport  Port=2
  Fy : Inport  Port=3
  CK_Factor : Inport  Port=4
  Kamm_Circle LatD : MATLAB Function  TreatAsAtomicUnit=on
  Product1 : Product
  Product2 : Product
  Fx_R : Outport  VectorParamsAs1DForOutWhenUnconnected=off
  Fx_L : Outport  Port=2  VectorParamsAs1DForOutWhenUnconnected=off
  Fy_R [N] (0,inf) : Outport  Port=3  VectorParamsAs1DForOutWhenUnconnected=off
  wires:
  Kamm_Circle LatD/3(Fy_R) -> Fy_R [N] (0,inf)/1
  Fz_L/1 -> Kamm_Circle LatD/2(Fz_L)
  Fz_R/1 -> Kamm_Circle LatD/1(Fz_R)
  Fy/1 -> Kamm_Circle LatD/3(Fy)
  Kamm_Circle LatD/1(Fx_R) -> Product1/1
  Kamm_Circle LatD/2(Fx_L) -> Product2/1
  Product2/1 -> Fx_L/1
  CK_Factor/1 -> Product2/2, Product1/2
  Product1/1 -> Fx_R/1

== system OPENXWD/CarMaker/IPG Vehicle/PowerTrain/Electric Powertrain/E-Gas // E-Motor/Subsystem1/VDC/Vehicle Dynamics Control Modes/VDC Complete/Lateral Dynamics/Tire Longitudinal Force Difference ==
  e : Inport
  Iz : Inport  Port=2
  dt : Inport  Port=3
  rt : Inport  Port=4
  " Momentum_Z to Longitudinal Force Difference" : Subsystem
  Momentum respect to Z-axis to correct the error : Subsystem
  Scope5 : Scope
  Scope6 : Scope
  Fx_diff : Outport  VectorParamsAs1DForOutWhenUnconnected=off
  wires:
  dt/1 -> Momentum respect to Z-axis to correct the error/3(Correction_Time [s])
  rt/1 -> " Momentum_Z to Longitudinal Force Difference"/2(RearTrackwidth [m])
  " Momentum_Z to Longitudinal Force Difference"/1(Fx_diff [N]) -> Fx_diff/1
  Iz/1 -> Momentum respect to Z-axis to correct the error/2(Iz [kg/m^3])
  Momentum respect to Z-axis to correct the error/1(Momentum_Z [Nm]) -> " Momentum_Z to Longitudinal Force Difference"/1("\tMomentumZ [Nm]"), Scope6/1
  e/1 -> Scope5/1, Momentum respect to Z-axis to correct the error/1(Yaw_error_[º/s])

== system OPENXWD/CarMaker/IPG Vehicle/PowerTrain/Electric Powertrain/E-Gas // E-Motor/Subsystem1/VDC/Vehicle Dynamics Control Modes/VDC Complete/Lateral Dynamics/Yaw_Rate_Reference ==
  Steering_Angle : Inport
  F_vel_x : Inport  Port=2
  360/(2*pi) : Gain  Gain=360/(2*pi)
  360/(2pi) : Gain  Gain=360/(2*pi)
  Bicycle Model : MATLAB Function  TreatAsAtomicUnit=on
  Constant7 : Constant  Value=0.92
  Constant8 : Constant  Value=360
  Cornering_Stiffness_F[N/º] : Constant  Value=-700
  Cornering_Stiffness_R[N/º] : Constant  Value=-1000
  Divide : Product  Inputs=*/
  Gain{,1..4} (5 alike) : Gain  Gain=360/(2*pi)
  Scope1 : Scope  NumInputPorts=5
  Scope2 : Scope  NumInputPorts=2
  Scope3 : Scope
  Steering_Ratio [-] : Constant  Value=3.72
  Wheelbase [m] : Constant  Value=1.53
  Yaw_Rate : Outport  VectorParamsAs1DForOutWhenUnconnected=off
  wires:
  Gain4/1 -> Scope1/2
  Gain3/1 -> Scope1/3
  Gain2/1 -> Scope1/4
  Gain1/1 -> Scope1/1
  Gain/1 -> Scope1/5
  360/(2pi)/1 -> Bicycle Model/7(cr)
  Cornering_Stiffness_R[N/º]/1 -> 360/(2pi)/1
  360/(2*pi)/1 -> Bicycle Model/6(cf)
  Bicycle Model/2(beta) -> Gain2/1
  F_vel_x/1 -> Bicycle Model/2(vx)
  Bicycle Model/7(yf) -> Scope2/1
  Bicycle Model/3(alpha_f) -> Gain4/1
  Bicycle Model/6(radius) -> Scope3/1
  Cornering_Stiffness_F[N/º]/1 -> 360/(2*pi)/1
  Constant7/1 -> Bicycle Model/4(xCG)
  Bicycle Model/5(course) -> Gain/1
  Constant8/1 -> Bicycle Model/3(m)
  Bicycle Model/4(alpha_r) -> Gain3/1
  Steering_Ratio [-]/1 -> Divide/2
  Bicycle Model/1(r) -> Yaw_Rate/1
  Divide/1 -> Gain1/1, Bicycle Model/1(delta)
  Wheelbase [m]/1 -> Bicycle Model/5(L)
  Steering_Angle/1 -> Divide/1
  Bicycle Model/8(yr) -> Scope2/2

== system OPENXWD/CarMaker/IPG Vehicle/PowerTrain/Electric Powertrain/E-Gas // E-Motor/Subsystem1/VDC/Vehicle Dynamics Control Modes/VDC Complete/Longitudinal Dynamics/Kamm_Circle ==
  Fz_R : Inport
  Fz_L : Inport  Port=2
  Fy : Inport  Port=3
  SK_Factor : Inport  Port=4
  Kamm_Circle LatD : MATLAB Function  TreatAsAtomicUnit=on
  Product : Product
  Product1 : Product
  Fx_R : Outport  VectorParamsAs1DForOutWhenUnconnected=off
  Fx_L : Outport  Port=2  VectorParamsAs1DForOutWhenUnconnected=off
  wires:
  Kamm_Circle LatD/1(Fx_R) -> Product/1
  Kamm_Circle LatD/2(Fx_L) -> Product1/1
  Fz_L/1 -> Kamm_Circle LatD/2(Fz_L)
  Fy/1 -> Kamm_Circle LatD/3(Fy)
  SK_Factor/1 -> Product/2, Product1/2
  Product/1 -> Fx_R/1
  Product1/1 -> Fx_L/1
  Fz_R/1 -> Kamm_Circle LatD/1(Fz_R)

== system OPENXWD/CarMaker/IPG Vehicle/PowerTrain/Electric Powertrain/E-Gas // E-Motor/Subsystem1/VDC/Vehicle Dynamics Control Modes/VDC Complete/Optimization SKF & CKF/Subsystem  ==
  Steer_An : Inport
  Derivative : Inport  Port=2
  SKF_Initial : Inport  Port=3
  SKF_prev : Inport  Port=4
  "CKF_Initial " : Inport  Port=5
  "CKF_prev " : Inport  Port=6
  Cte_SKF : Inport  Port=7
  Cte_CKF : Inport  Port=8
  CKF : Subsystem
  MATLAB Function1 : MATLAB Function  TreatAsAtomicUnit=on
  SKF : Subsystem
  SKF or CKF : If  IfExpression=-10 < u1 & u1 < 10
  Steering Wheel Maximum Angle : Constant  Value=100
  "SKF_act " : Outport  VectorParamsAs1DForOutWhenUnconnected=off
  CKF_act : Outport  Port=2  VectorParamsAs1DForOutWhenUnconnected=off
  wires:
  MATLAB Function1/1(value) -> SKF or CKF/1
  Steering Wheel Maximum Angle/1 -> MATLAB Function1/1(cte)
  Steer_An/1 -> MATLAB Function1/2(v)
  SKF/1(SKF_act) -> "SKF_act "/1
  CKF/1("CKF_act ") -> CKF_act/1
  SKF or CKF/1 -> SKF/Action
  SKF or CKF/2 -> CKF/Action
  "CKF_prev "/1 -> CKF/3("CKF_prev ")
  Derivative/1 -> CKF/1(Derivative), SKF/1(Derivative)
  SKF_Initial/1 -> SKF/2("SKF_Initial ")
  SKF_prev/1 -> SKF/3(SKF_prev)
  "CKF_Initial "/1 -> CKF/2(CKF_Initial)
  Cte_SKF/1 -> SKF/4(Cte_SKF)
  Cte_CKF/1 -> CKF/4(Cte_CKF)

== system OPENXWD/CarMaker/IPG Vehicle/PowerTrain/Electric Powertrain/E-Gas // E-Motor/Subsystem1/VDC/Vehicle Dynamics Control Modes/VDC Complete/Wheel_to_motor/Fx_to_engineTqRL ==
  Fx : Inport
  Re : Inport  Port=2
  RT : Inport  Port=3
  Divide : Product  Inputs=*/
  Product : Product
  Tq : Outport  VectorParamsAs1DForOutWhenUnconnected=off
  wires:
  Divide/1 -> Tq/1
  Product/1 -> Divide/1
  RT/1 -> Divide/2
  Fx/1 -> Product/1
  Re/1 -> Product/2

== system OPENXWD/CarMaker/IPG Vehicle/PowerTrain/Electric Powertrain/E-Gas // E-Motor/Subsystem1/VDC/Vehicle Dynamics Control Modes/VDC Complete/Wheel_to_motor/Fx_to_engineTqRR ==
  Fx : Inport
  Re : Inport  Port=2
  RT : Inport  Port=3
  Divide : Product  Inputs=*/
  Product : Product
  Tq : Outport  VectorParamsAs1DForOutWhenUnconnected=off
  wires:
  Divide/1 -> Tq/1
  Product/1 -> Divide/1
  RT/1 -> Divide/2
  Fx/1 -> Product/1
  Re/1 -> Product/2

== system OPENXWD/CarMaker/IPG Vehicle/PowerTrain/Electric Powertrain/E-Gas // E-Motor/Subsystem1/VDC/Vehicle Dynamics Control Modes/VDC without Longitudinal/Constraints/Acelerating and braking without Regenerative ==
  Transmission Ratio : Inport
  Tq_max : Inport  Port=2
  V_eRR : Inport  Port=3
  V_eRL : Inport  Port=4
  Trans_dynamic_max_motor_Tq : Inport  Port=5
  Trans_static_max_motor_Tq : Inport  Port=6
  Tq_FR : Inport  Port=7
  Tq_FL : Inport  Port=8
  Tq_RR : Inport  Port=9
  Tq_RL : Inport  Port=10
  Action Port : ActionPort  ActionPortLabel=else
  Gain : Gain  Gain=3.141592/30
  If Action 1 : Subsystem  TreatAsAtomicUnit=on
  If Action 2 : Subsystem  TreatAsAtomicUnit=on
  If1 : If  NumInputs=3  IfExpression=u1 > u3 & u2 > u3
  Merge2 : Merge
  Momentum Z scaled : Subsystem
  Terminator : Terminator
  Terminator1 : Terminator
  To wheel Tq (dynamic) : Product
  To wheel Tq (static) : Product
  minimum value : MATLAB Function  TreatAsAtomicUnit=on
  minimum value1 : MATLAB Function  TreatAsAtomicUnit=on
  rpm : Constant  Value=200
  TQ_RR : Outport  VectorParamsAs1DForOutWhenUnconnected=off
  TQ_RL : Outport  Port=2  VectorParamsAs1DForOutWhenUnconnected=off
  wires:
  If1/1 -> If Action 1/Action
  If Action 1/1(Trans_limit) -> Merge2/1
  Merge2/1 -> minimum value/1(a), minimum value1/1(a)
  If Action 2/1(Trans_limit) -> Merge2/2
  V_eRR/1 -> If1/1
  V_eRL/1 -> If1/2
  If1/2 -> If Action 2/Action
  Tq_max/1 -> minimum value1/2(b), minimum value/2(b)
  rpm/1 -> Gain/1
  Gain/1 -> If1/3  "approx 20.95"
  Tq_FR/1 -> Terminator/1
  Tq_FL/1 -> Terminator1/1
  Tq_RR/1 -> [tq_RR_wc], minimum value/3(c)
  Tq_RL/1 -> [tq_RL_wc], minimum value1/3(c)
  [tq_RR_wc] -> Momentum Z scaled/3(Tq_RR_wc)
  [tq_RL_wc] -> Momentum Z scaled/4(Tq_RL_wc)
  Momentum Z scaled/1(TQ_RR) -> TQ_RR/1
  Momentum Z scaled/2(TQ_RL) -> TQ_RL/1
  minimum value1/1(min) -> Momentum Z scaled/2(Tq_RL_Lim)
  minimum value/1(min) -> Momentum Z scaled/1(Tq_RR_Lim)
  Trans_dynamic_max_motor_Tq/1 -> To wheel Tq (dynamic)/1
  Transmission Ratio/1 -> To wheel Tq (static)/1, To wheel Tq (dynamic)/2
  Trans_static_max_motor_Tq/1 -> To wheel Tq (static)/2
  To wheel Tq (static)/1 -> If Action 2/1("Trans_max_static ")
  To wheel Tq (dynamic)/1 -> If Action 1/1(Trans_max_dynamic)

== system OPENXWD/CarMaker/IPG Vehicle/PowerTrain/Electric Powertrain/E-Gas // E-Motor/Subsystem1/VDC/Vehicle Dynamics Control Modes/VDC without Longitudinal/Constraints/Braking with Regenerative ==
  MaxRegTorque : Inport
  Tq_RR_wc : Inport  Port=2
  Tq_RL_wc : Inport  Port=3
  Action Port : ActionPort  ActionPortLabel=if(u2 == 1 & u1 > 0)
  Gain : Gain  Gain=-1
  Gain1 : Gain  Gain=-1
  MATLAB Function : MATLAB Function  TreatAsAtomicUnit=on
  TQ_RR : Outport  VectorParamsAs1DForOutWhenUnconnected=off
  TQ_RL : Outport  Port=2  VectorParamsAs1DForOutWhenUnconnected=off
  wires:
  MaxRegTorque/1 -> MATLAB Function/1(MaxRegenTq)
  Gain1/1 -> TQ_RL/1
  Gain/1 -> TQ_RR/1
  Tq_RL_wc/1 -> MATLAB Function/3(Tq_RL)
  Tq_RR_wc/1 -> MATLAB Function/2(Tq_RR)
  MATLAB Function/1(RegTq_RR) -> Gain/1
  MATLAB Function/2(RegTq_RL) -> Gain1/1

== system OPENXWD/CarMaker/IPG Vehicle/PowerTrain/Electric Powertrain/E-Gas // E-Motor/Subsystem1/VDC/Vehicle Dynamics Control Modes/VDC without Longitudinal/Driver // CarBehaviours/Accelerating ==
  Ap : Inport
  "Ap_Sat_up " : Inport  Port=2
  Ap_Sat_down : Inport  Port=3
  Tq_RR : Inport  Port=4
  "Tq_RL " : Inport  Port=5
  Action Port : ActionPort  ActionPortLabel=else
  "Accelerator behaviour " : MATLAB Function  TreatAsAtomicUnit=on
  Product : Product
  Product1 : Product
  "Tq_RR " : Outport  VectorParamsAs1DForOutWhenUnconnected=off
  Tq_RL : Outport  Port=2  VectorParamsAs1DForOutWhenUnconnected=off
  Out_Throttle : Outport  Port=3  VectorParamsAs1DForOutWhenUnconnected=off
  wires:
  Ap/1 -> "Accelerator behaviour "/1(Ap)
  "Ap_Sat_up "/1 -> "Accelerator behaviour "/2(Ap_Sat_up)
  Ap_Sat_down/1 -> "Accelerator behaviour "/3(Ap_Sat_down)
  Product1/1 -> "Tq_RR "/1
  Product/1 -> Tq_RL/1
  "Accelerator behaviour "/1(throttle) -> Out_Throttle/1, Product/1, Product1/1
  Tq_RR/1 -> Product1/2
  "Tq_RL "/1 -> Product/2

== system OPENXWD/CarMaker/IPG Vehicle/PowerTrain/Electric Powertrain/E-Gas // E-Motor/Subsystem1/VDC/Vehicle Dynamics Control Modes/VDC without Longitudinal/Driver // CarBehaviours/Inertia Braking ==
  Action Port : ActionPort  ActionPortLabel=elseif( u1==0 & u2==0)
  Constant : Constant  Value=0
  Constant1 : Constant  Value=0
  "Tq_RR " : Outport  VectorParamsAs1DForOutWhenUnconnected=off
  Tq_RL : Outport  Port=2  VectorParamsAs1DForOutWhenUnconnected=off
  wires:
  Constant1/1 -> Tq_RL/1
  Constant/1 -> "Tq_RR "/1

== system OPENXWD/CarMaker/IPG Vehicle/PowerTrain/Electric Powertrain/E-Gas // E-Motor/Subsystem1/VDC/Vehicle Dynamics Control Modes/VDC without Longitudinal/Driver // CarBehaviours/Mech_Braking ==
  Action Port : ActionPort  ActionPortLabel=elseif(u1>0.2 & u2<=u4 & u3==0)
  Constant : Constant  Value=0
  Constant1 : Constant  Value=0
  "Tq_RR " : Outport  VectorParamsAs1DForOutWhenUnconnected=off
  Tq_RL : Outport  Port=2  VectorParamsAs1DForOutWhenUnconnected=off
  wires:
  Constant1/1 -> Tq_RL/1
  Constant/1 -> "Tq_RR "/1

== system OPENXWD/CarMaker/IPG Vehicle/PowerTrain/Electric Powertrain/E-Gas // E-Motor/Subsystem1/VDC/Vehicle Dynamics Control Modes/VDC without Longitudinal/Driver // CarBehaviours/Regenerative+Mech Braking ==
  Bp : Inport
  Tq_max_RR : Inport  Port=2
  Tq_max_RL : Inport  Port=3
  Action Port : ActionPort  ActionPortLabel=if(u1>0.2 & u2<=u4 & u3==1)
  MATLAB Function : MATLAB Function  TreatAsAtomicUnit=on
  "Tq_RR " : Outport  VectorParamsAs1DForOutWhenUnconnected=off
  Tq_RL : Outport  Port=2  VectorParamsAs1DForOutWhenUnconnected=off
  wires:
  Bp/1 -> MATLAB Function/1(Bp)
  Tq_max_RR/1 -> MATLAB Function/2(Tq_max_RR)
  Tq_max_RL/1 -> MATLAB Function/3(Tq_max_RL)
  MATLAB Function/1(Tq_regen_RR) -> "Tq_RR "/1
  MATLAB Function/2(Tq_regen_RL) -> Tq_RL/1

== system OPENXWD/CarMaker/IPG Vehicle/PowerTrain/Electric Powertrain/E-Gas // E-Motor/Subsystem1/VDC/Vehicle Dynamics Control Modes/VDC without Longitudinal/Force to Tq/Fx_to_wheelTqRL ==
  Fx : Inport
  Re : Inport  Port=2
  Product : Product
  Tq : Outport  VectorParamsAs1DForOutWhenUnconnected=off
  wires:
  Product/1 -> Tq/1
  Fx/1 -> Product/1
  Re/1 -> Product/2

== system OPENXWD/CarMaker/IPG Vehicle/PowerTrain/Electric Powertrain/E-Gas // E-Motor/Subsystem1/VDC/Vehicle Dynamics Control Modes/VDC without Longitudinal/Force to Tq/Fx_to_wheelTqRR ==
  Fx : Inport
  Re : Inport  Port=2
  Product : Product
  Tq : Outport  VectorParamsAs1DForOutWhenUnconnected=off
  wires:
  Product/1 -> Tq/1
  Fx/1 -> Product/1
  Re/1 -> Product/2

== system OPENXWD/CarMaker/IPG Vehicle/PowerTrain/Electric Powertrain/E-Gas // E-Motor/Subsystem1/VDC/Vehicle Dynamics Control Modes/VDC without Longitudinal/Optimization SKF & CKF/Subsystem  ==
  Derivative : Inport
  "CKF_Initial " : Inport  Port=2
  "CKF_prev " : Inport  Port=3
  Cte_CKF : Inport  Port=4
  CKF : Subsystem
  CKF_act : Outport  VectorParamsAs1DForOutWhenUnconnected=off
  wires:
  CKF/1("CKF_act ") -> CKF_act/1
  "CKF_prev "/1 -> CKF/3("CKF_prev ")
  Derivative/1 -> CKF/1(Derivative)
  "CKF_Initial "/1 -> CKF/2(CKF_Initial)
  Cte_CKF/1 -> CKF/4(Cte_CKF)

== system OPENXWD/CarMaker/IPG Vehicle/PowerTrain/Electric Powertrain/E-Gas // E-Motor/Subsystem1/VDC/Vehicle Dynamics Control Modes/Steering TV with TC/Optimization SKF & CKF/Subsystem /CKF ==
  Derivative : Inport
  CKF_Initial : Inport  Port=2
  "CKF_prev " : Inport  Port=3
  Cte_CKF : Inport  Port=4
  Action Port : ActionPort  ActionPortLabel=else
  If1 : If  IfExpression=u1 >= 900  ElseIfExpressions=u1 < 900  ShowElse=off
  Merge : Merge
  No spin : Subsystem  TreatAsAtomicUnit=on
  Saturation : Saturate  UpperLimit=1  LowerLimit=0.3
  "Spin " : Subsystem  TreatAsAtomicUnit=on
  "CKF_act " : Outport  VectorParamsAs1DForOutWhenUnconnected=off
  wires:
  Merge/1 -> Saturation/1
  "CKF_prev "/1 -> "Spin "/1(CKF_prev), No spin/2(CKF_prev)
  If1/1 -> "Spin "/Action
  Cte_CKF/1 -> No spin/3(Cte_CKF), "Spin "/3(Cte_CKF)
  "Spin "/1("CKF_act1 ") -> Merge/2
  Saturation/1 -> "CKF_act "/1
  CKF_Initial/1 -> "Spin "/2("CKF_Initial "), No spin/1(CKF_Initial)
  If1/2 -> No spin/Action
  No spin/1(CKF_act0) -> Merge/1
  Derivative/1 -> If1/1

== system OPENXWD/CarMaker/IPG Vehicle/PowerTrain/Electric Powertrain/E-Gas // E-Motor/Subsystem1/VDC/Vehicle Dynamics Control Modes/Steering TV with TC/Optimization SKF & CKF/Subsystem /SKF ==
  Derivative : Inport
  "SKF_Initial " : Inport  Port=2
  SKF_prev : Inport  Port=3
  Cte_SKF : Inport  Port=4
  Action Port : ActionPort  ActionPortLabel=if(-10 < u1 & u1 < 10)
  Display1 : Display
  If : If  IfExpression=u1 >=900  ElseIfExpressions=u1 < 900  ShowElse=off
  Merge : Merge
  No spin : Subsystem  TreatAsAtomicUnit=on
  Saturation : Saturate  UpperLimit=1  LowerLimit=0.3
  Spin : Subsystem  TreatAsAtomicUnit=on
  SKF_act : Outport  VectorParamsAs1DForOutWhenUnconnected=off
  wires:
  Merge/1 -> Saturation/1
  Spin/1(SKF_act1) -> Merge/2
  "SKF_Initial "/1 -> Spin/1(SKF_Initial), No spin/1(SKF_Initial)
  No spin/1(SKF_act0) -> Merge/1
  If/2 -> No spin/Action
  SKF_prev/1 -> No spin/2(SKF_prev), Spin/2(SKF_prev)
  Saturation/1 -> Display1/1, SKF_act/1
  If/1 -> Spin/Action
  Derivative/1 -> If/1
  Cte_SKF/1 -> Spin/3(Cte_SKF), No spin/3(Cte_SKF)

== system OPENXWD/CarMaker/IPG Vehicle/PowerTrain/Electric Powertrain/E-Gas // E-Motor/Subsystem1/VDC/Vehicle Dynamics Control Modes/VDC Complete/Constraints and motor to wheel Tq/Acelerating and braking without Regenerative/If Action 1 ==
  Trans_max_dynamic : Inport
  Action Port : ActionPort  ActionPortLabel=if(u1 > u3 & u2 > u3)
  Trans_limit : Outport  VectorParamsAs1DForOutWhenUnconnected=off
  wires:
  Trans_max_dynamic/1 -> Trans_limit/1

== system OPENXWD/CarMaker/IPG Vehicle/PowerTrain/Electric Powertrain/E-Gas // E-Motor/Subsystem1/VDC/Vehicle Dynamics Control Modes/VDC Complete/Constraints and motor to wheel Tq/Acelerating and braking without Regenerative/If Action 2 ==
  "Trans_max_static " : Inport
  Action Port : ActionPort  ActionPortLabel=else
  Trans_limit : Outport  VectorParamsAs1DForOutWhenUnconnected=off
  wires:
  "Trans_max_static "/1 -> Trans_limit/1

== system OPENXWD/CarMaker/IPG Vehicle/PowerTrain/Electric Powertrain/E-Gas // E-Motor/Subsystem1/VDC/Vehicle Dynamics Control Modes/VDC Complete/Constraints and motor to wheel Tq/Acelerating and braking without Regenerative/Momentum Z scaled ==
  Tq_RR_Lim : Inport
  Tq_RL_Lim : Inport  Port=2
  Tq_RR_wc : Inport  Port=3
  Tq_RL_wc : Inport  Port=4
  Tq_diff : Inport  Port=5
  Display : Display
  Display1 : Display
  MATLAB Function : MATLAB Function  TreatAsAtomicUnit=on
  TQ_RR : Outport  VectorParamsAs1DForOutWhenUnconnected=off
  TQ_RL : Outport  Port=2  VectorParamsAs1DForOutWhenUnconnected=off
  wires:
  Tq_RL_Lim/1 -> MATLAB Function/2(tq_RL_lim)
  Tq_RR_Lim/1 -> MATLAB Function/1(tq_RR_lim)
  Tq_RR_wc/1 -> MATLAB Function/3(tq_RR_wc)
  Tq_RL_wc/1 -> MATLAB Function/4(tq_RL_wc)
  MATLAB Function/1(TQ_RR) -> Display/1, TQ_RR/1
  MATLAB Function/2(TQ_RL) -> Display1/1, TQ_RL/1
  Tq_diff/1 -> MATLAB Function/5(tq_diff)

== system OPENXWD/CarMaker/IPG Vehicle/PowerTrain/Electric Powertrain/E-Gas // E-Motor/Subsystem1/VDC/Vehicle Dynamics Control Modes/VDC Complete/Lateral Dynamics/Tire Longitudinal Force Difference/ Momentum_Z to Longitudinal Force Difference ==
  "\tMomentumZ [Nm]" : Inport
  RearTrackwidth [m] : Inport  Port=2
  Constant : Constant  Value=2
  Divide : Product  Inputs=*/
  Divide1 : Product  Inputs=*/
  Fx_diff [N] : Outport  VectorParamsAs1DForOutWhenUnconnected=off
  wires:
  Divide/1 -> Fx_diff [N]/1
  Divide1/1 -> Divide/2
  "\tMomentumZ [Nm]"/1 -> Divide/1
  Constant/1 -> Divide1/2
  RearTrackwidth [m]/1 -> Divide1/1
